simulink model "Modello_carroponte_non_lin"  (R2024a)
settings: Solver=FixedStepAuto  StartTime=tempo(1)  StopTime=tempo(end)  FixedStep=dt  RelTol=1e-3
undefined symbols (not defined in the file): alpha_0, alpha_dot_0, cc, cm, dinamica_alpha, g, L, mc, mm, xc_0, xc_dot_0
settings Model: Creator=smila  LastModifiedBy=smila
settings OptimizationCC: BlockReduction=off  DefaultParameterBehavior=Inlined  BufferReuse=off

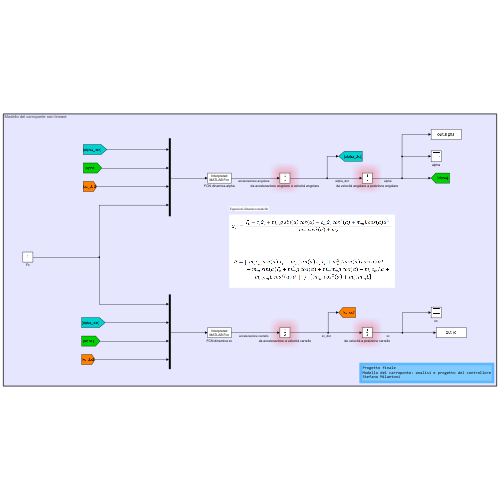
[thumbnail: Simulink's stored preview of the top-level diagram]
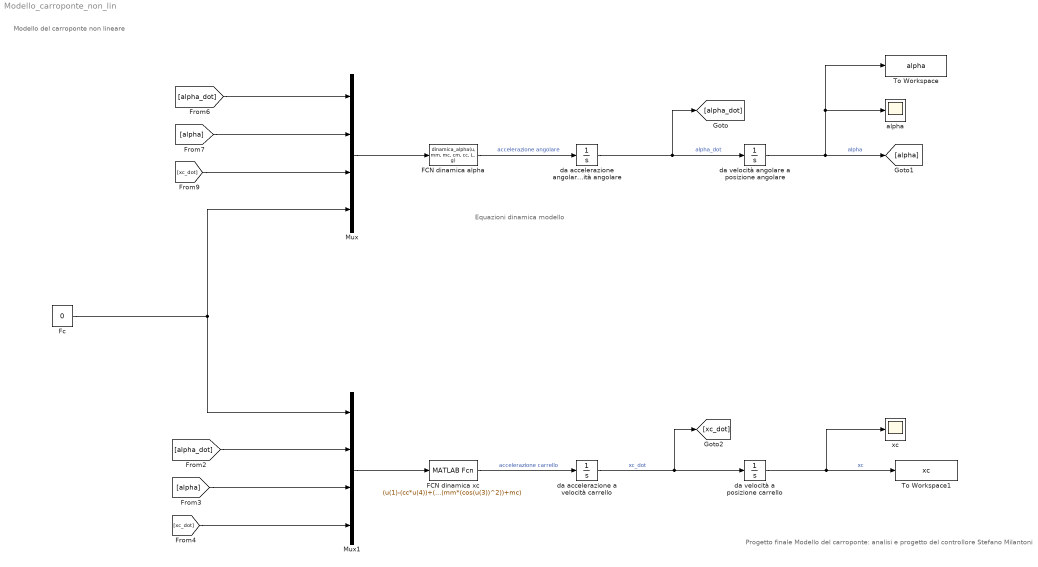
== system Modello_carroponte_non_lin ==
  note: Equazioni dinamica modello
  note: Progetto finale
      | Modello del carroponte: analisi e progetto del controllore
      | Stefano Milantoni
  note: Modello del carroponte non lineare
  FCN dinamica alpha : MATLABFcn  MATLABFcn=dinamica_alpha(u, mm, mc, cm, cc, L, g)
  FCN dinamica xc : MATLABFcn  MATLABFcn=(u(1)-(cc*u(4))+(mm*g*sin(u(3))*cos(u(3)))-(cm*u(4)*(cos(u(3))^2))+(mm*L*cos(u(3))*(u(2)^2)))/((mm*(cos(u(3))^2))+mc)
  Fc : Constant  Value=0
  Mux : Mux
  Mux1 : Mux
  To Workspace : ToWorkspace  VariableName=alpha  SampleTime=-1
  To Workspace1 : ToWorkspace  VariableName=xc  SampleTime=-1
  alpha : Scope
  da accelerazione a velocità carrello : Integrator  InitialCondition=xc_dot_0
  da accelerazione angolare a velocità angolare : Integrator  InitialCondition=alpha_dot_0
  da velocità a posizione carrello : Integrator  InitialCondition=xc_0
  da velocità angolare a posizione angolare : Integrator  InitialCondition=alpha_0
  xc : Scope
  wires:
  [alpha] -> Mux1/3
  FCN dinamica xc/1 -> da accelerazione a velocità carrello/1  "accelerazione carrello"
  [xc_dot] -> Mux1/4
  da velocità a posizione carrello/1 -> xc/1, To Workspace1/1  "xc"
  Mux1/1 -> FCN dinamica xc/1
  da accelerazione a velocità carrello/1 -> da velocità a posizione carrello/1, [xc_dot]  "xc_dot"
  Mux/1 -> FCN dinamica alpha/1
  da velocità angolare a posizione angolare/1 -> To Workspace/1, alpha/1, [alpha]  "alpha"
  [alpha_dot] -> Mux/1
  [alpha_dot] -> Mux1/2
  Fc/1 -> Mux/4, Mux1/1
  da accelerazione angolare a velocità angolare/1 -> da velocità angolare a posizione angolare/1, [alpha_dot]  "alpha_dot"
  [xc_dot] -> Mux/3
  [alpha] -> Mux/2
  FCN dinamica alpha/1 -> da accelerazione angolare a velocità angolare/1  "accelerazione angolare"
